simulink model "Simulink_model"  (R2024b)
settings: Solver=FixedStepAuto  StartTime=0.0  StopTime=10.0  FixedStep=1e-3  RelTol=1e-3
undefined symbols (not defined in the file): G, K, Nu, Nx, T_L
settings Model: Creator=Enrico  LastModifiedBy=Enrico

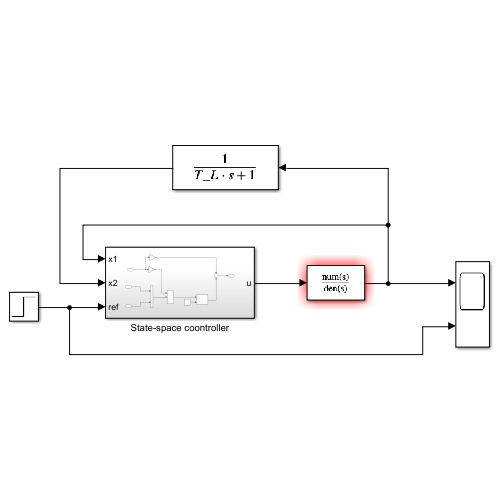
[thumbnail: Simulink's stored preview of the top-level diagram]
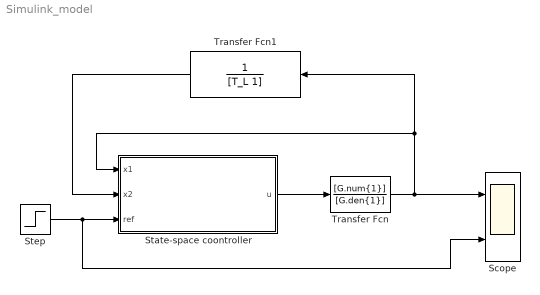
== system Simulink_model ==
  Scope : Scope  NumInputPorts=2
  State-space coontroller : Subsystem
  Step : Step  SampleTime=0
  Transfer Fcn : TransferFcn  Numerator=[G.num{1}]  Denominator=[G.den{1}]
  Transfer Fcn1 : TransferFcn  Denominator=[T_L 1]
  wires:
  State-space coontroller/1(u) -> Transfer Fcn/1
  Transfer Fcn/1 -> Scope/1, Transfer Fcn1/1, State-space coontroller/1(x1)
  Transfer Fcn1/1 -> State-space coontroller/2(x2)
  Step/1 -> Scope/2, State-space coontroller/3(ref)

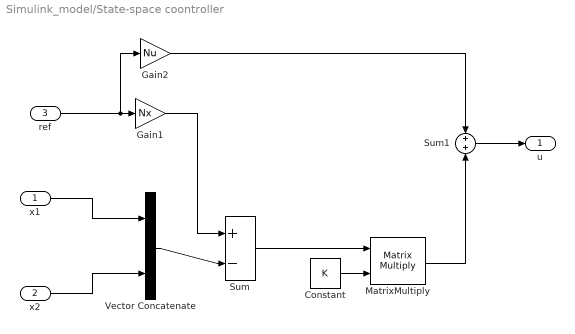
== system Simulink_model/State-space coontroller ==
  x1 : Inport
  x2 : Inport  Port=2
  ref : Inport  Port=3
  Constant : Constant  Value=K
  Gain1 : Gain  Gain=Nx
  Gain2 : Gain  Gain=Nu
  MatrixMultiply : Product  Multiplication=Matrix(*)
  Sum : Sum  Inputs=+-|
  Sum1 : Sum  Inputs=+|+
  Vector Concatenate : Concatenate
  u : Outport
  wires:
  x2/1 -> Vector Concatenate/2
  Constant/1 -> MatrixMultiply/2
  x1/1 -> Vector Concatenate/1
  Vector Concatenate/1 -> Sum/2
  Gain1/1 -> Sum/1
  ref/1 -> Gain2/1, Gain1/1
  Sum/1 -> MatrixMultiply/1
  MatrixMultiply/1 -> Sum1/2
  Gain2/1 -> Sum1/1
  Sum1/1 -> u/1
